simulink model "lab_04_03"  (R2024b)
settings: Solver=VariableStepAuto  StartTime=0.0  StopTime=10.0  RelTol=1e-3

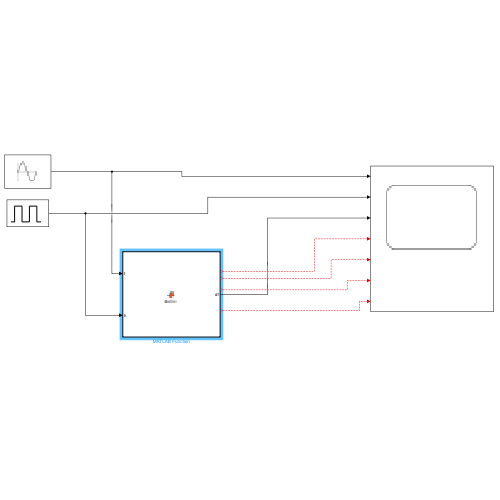
[thumbnail: Simulink's stored preview of the top-level diagram]
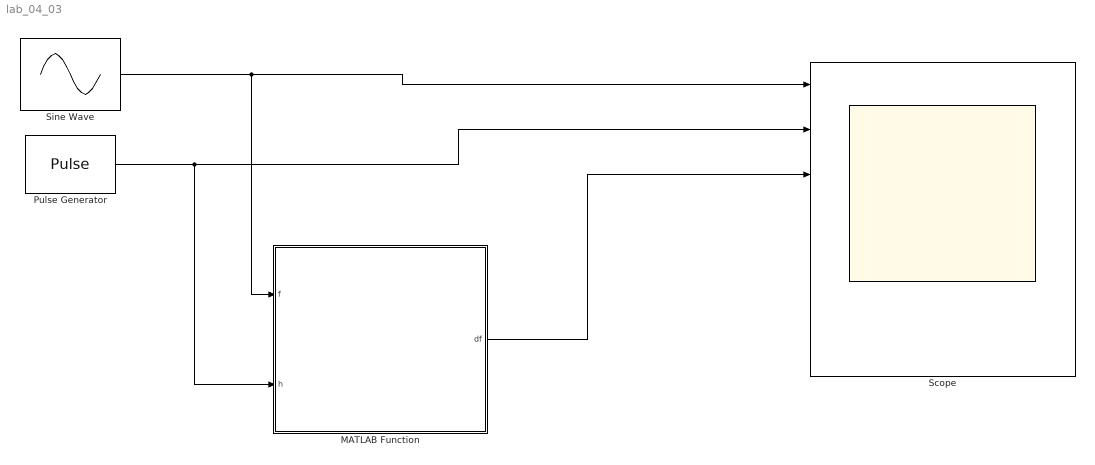
== system lab_04_03 ==
  MATLAB Function : MATLAB Function  TreatAsAtomicUnit=on
  Pulse Generator : DiscretePulseGenerator  PulseType=Time based  Amplitude=10  PulseWidth=6
  Scope : Scope  NumInputPorts=7
  Sine Wave : Sin  SampleTime=0
  wires:
  Pulse Generator/1 -> MATLAB Function/2(h), Scope/2
  Sine Wave/1 -> Scope/1, MATLAB Function/1(f)
  MATLAB Function/1(df) -> Scope/3
  ? -> Scope/4
  ? -> Scope/5
  ? -> Scope/6
  ? -> Scope/7

== matlab function lab_04_03/MATLAB Function ==
  data: f input; df output; h input

%function df = deriv(f,a,h)

%df(a) = (f(a+h)-f(a-h))/(2*h);

%end

function df =  deriv(f,h) 

    n = length(f);
    df = zeros(size(f));

    df(1) = (f(2)-f(1))/h;

    for i = 2:n-1
        df(i) = (f(i+1) - f(i-1))/(2*h);
    end

    df(n) = (f(n) - f(n-1))/h
end

function [y1, y2, y3, y4, y5] = fcn(u1,u2)




%function [y1, y2, y3, y4, y5] = fcn(u1, u2, t)
%function [y1,y2,y3,y4,y5]= fcn(u1,u2,dt)

%y1 = conv(u1,u2);
%y2 = (u1+u2);
%y3 = (u1-u2);
%y4 = (u1.*u2);
%y5 = [diff(u1)/dt];


    y1 = conv(u1,u2);

    y2 = (u1+u2);

    y3 = (u1-u2);

    y4 = (u1.*u2);
    
    %h = 1;
    %y5 = [0,(u1(3:end) - u1(1:end-2))/(2*h),0];
    
    h = 0.01;

    y5 = deriv(u1,h);
    
end


%t = 0:0.1:2*pi;
%u1 = sin(t);

%[y1,y2,y3,y4,y5] = fcn(u1,u2,t);


%subplot(3,1,1);
%plot(t,u1);
%title('Sine wave (u1)');

%subplot(3,1,2);
%plot(t,y5);
%title('Derivative of u1 (y5)');

%subplot(3,1,3);
%plot(t,cos(t));
%title('Exact derivative cos(t)');
